simulink model "cdo_vawt_sil"  (R2025b)
settings: Solver=FixedStepDiscrete  StartTime=0  StopTime=31532400  FixedStep=3600  RelTol=1e-3
undefined symbols (not defined in the file or in its folder): matlab_vawt_sil_hour_step_vector
settings Model: Creator=User  LastModifiedBy=User

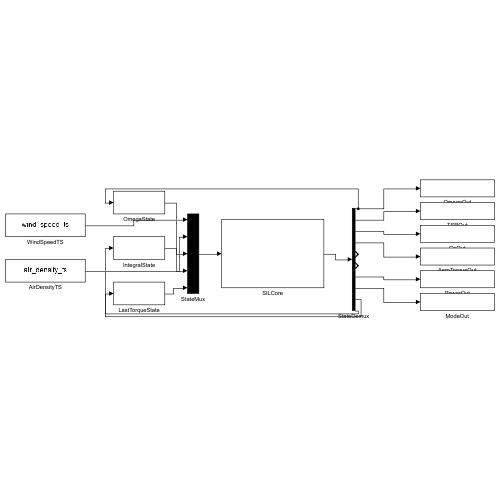
[thumbnail: Simulink's stored preview of the top-level diagram]
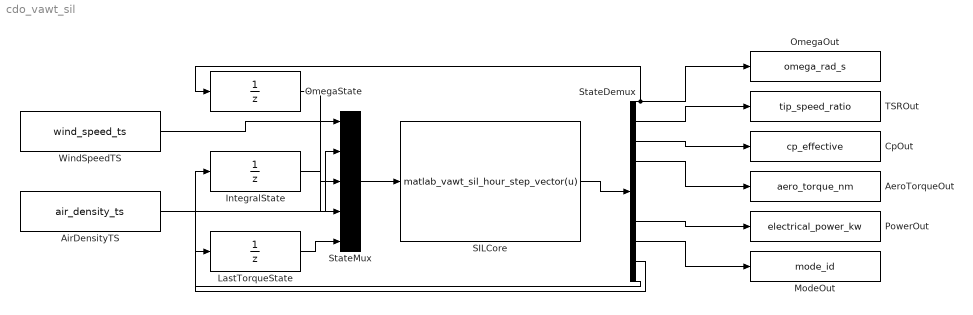
== system cdo_vawt_sil ==
  AeroTorqueOut : ToWorkspace  VariableName=aero_torque_nm  SaveFormat=Structure With Time  SampleTime=-1
  AirDensityTS : FromWorkspace  VariableName=air_density_ts
  CpOut : ToWorkspace  VariableName=cp_effective  SaveFormat=Structure With Time  SampleTime=-1
  IntegralState : UnitDelay  SampleTime=-1  HasFrameUpgradeWarning=on
  LastTorqueState : UnitDelay  SampleTime=-1  HasFrameUpgradeWarning=on
  ModeOut : ToWorkspace  VariableName=mode_id  SaveFormat=Structure With Time  SampleTime=-1
  OmegaOut : ToWorkspace  VariableName=omega_rad_s  SaveFormat=Structure With Time  SampleTime=-1
  OmegaState : UnitDelay  SampleTime=-1  HasFrameUpgradeWarning=on
  PowerOut : ToWorkspace  VariableName=electrical_power_kw  SaveFormat=Structure With Time  SampleTime=-1
  SILCore : MATLABFcn  MATLABFcn=matlab_vawt_sil_hour_step_vector(u)
  StateDemux : Demux  Outputs=10
  StateMux : Mux  Inputs=5
  TSROut : ToWorkspace  VariableName=tip_speed_ratio  SaveFormat=Structure With Time  SampleTime=-1
  WindSpeedTS : FromWorkspace  VariableName=wind_speed_ts
  wires:
  WindSpeedTS/1 -> StateMux/1
  AirDensityTS/1 -> StateMux/2
  OmegaState/1 -> StateMux/3
  IntegralState/1 -> StateMux/4
  LastTorqueState/1 -> StateMux/5
  StateMux/1 -> SILCore/1
  SILCore/1 -> StateDemux/1
  StateDemux/1 -> OmegaState/1, OmegaOut/1
  StateDemux/9 -> IntegralState/1
  StateDemux/10 -> LastTorqueState/1
  StateDemux/2 -> TSROut/1
  StateDemux/3 -> CpOut/1
  StateDemux/4 -> AeroTorqueOut/1
  StateDemux/7 -> PowerOut/1
  StateDemux/8 -> ModeOut/1
